simulink model "DiffDrive_Sim"  (R2022b)
settings: Solver=FixedStepAuto  StartTime=0.0  StopTime=120  FixedStep=Ts  RelTol=1e-3
values from neighbouring files (symbols this model uses):
  encoder_cpr = 12    [load_model.m]
  max_turning_radius = 100    [load_model.m]
  motor_FF_factor = 1.0    (= 1)    [load_model.m]
  motor_gear = 1/75    (= 0.0133333333333)    [load_model.m]
  motor_tf = load('..\data\platform\TF_motor.mat').TF_MOT    [load_model.m]
  motor_Ts = 50e-3    (= 0.05)    [load_model.m]
  motor_vcc = 5.93    [load_model.m]
  motor_vel_max = 47.5    [load_model.m]
  PID_mot_vel_coeff = get_PID_coeff(PID_mot_vel, motor_Ts)    [load_model.m]
  Ts = 1e-3    (= 0.001)    [load_model.m]
  wheel_radius = 0.01625    [load_model.m]
  wheel_track = 0.125/2    (= 0.0625)    [load_model.m]
libraries: cstblocks x2
settings Model: Creator=alexr  LastModifiedBy=alexr

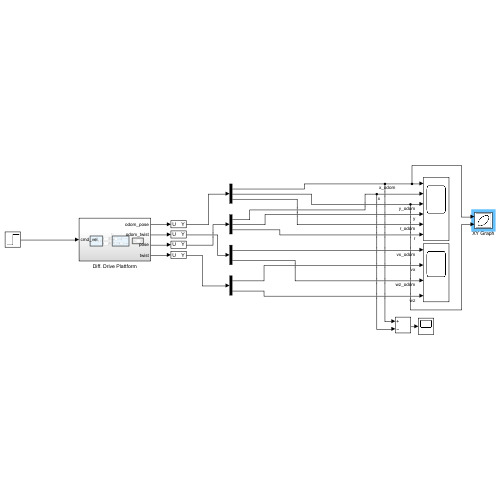
[thumbnail: Simulink's stored preview of the top-level diagram]
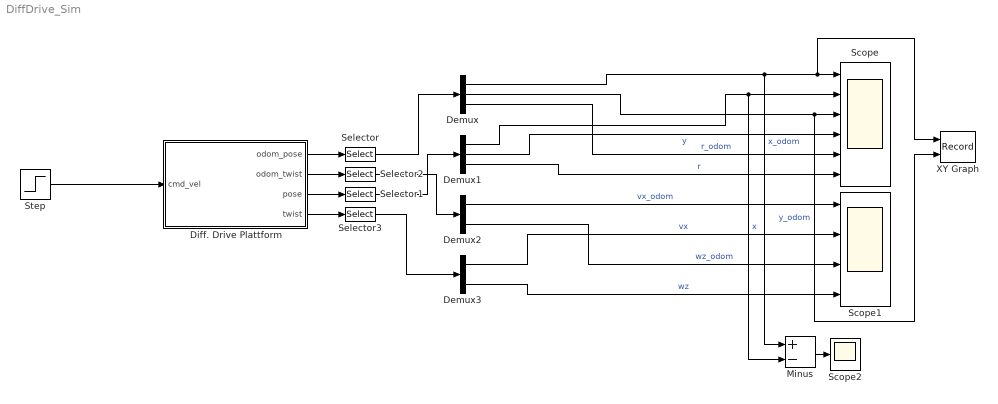
== system DiffDrive_Sim ==
  Demux : Demux  Outputs=3
  Demux1 : Demux  Outputs=3
  Demux2 : Demux  Outputs=2
  Demux3 : Demux  Outputs=2
  Diff. Drive Plattform : Subsystem
  Minus : Sum  Inputs=+-
  Scope : Scope  NumInputPorts=6
  Scope1 : Scope  NumInputPorts=4
  Scope2 : Scope
  Selector : Selector  InputPortWidth=6  IndexOptions=Index vector (dialog)  Indices=[1 2 6]  OutputSizes=1
  Selector1 : Selector  InputPortWidth=6  IndexOptions=Index vector (dialog)  Indices=[1 2 6]  OutputSizes=1
  Selector2 : Selector  InputPortWidth=6  IndexOptions=Index vector (dialog)  Indices=[1 6]  OutputSizes=1
  Selector3 : Selector  InputPortWidth=6  IndexOptions=Index vector (dialog)  Indices=[1 6]  OutputSizes=1
  Step : Step  After=[.1 0 0 0 0 .5]'  SampleTime=0
  XY Graph : Record  FileSettingsInternal="{\"entries\":[{\"content\":{\"excelSettings\":{\"content\":{},\"type\":\"Streamout.ExcelSettings\"}},\"type\":\"Streamout.FileSettingStorage\",\"uuid\":\"8a958047-305f-4305-a06c-71493970eef4\"}],\"packageUris\":[\"http://schema.mathworks.com/mf0/streamout_blocks/R2020a\"],\"version\":\"1.0\"}"  Layout=[1 1]  SignalsInternal="{\"entries\":[{\"content\":{\"signals\":[{\"content\":{\"blockPath\":[\"DiffDrive_Sim/XY Graph\"],\"channel\":[],\"dimensions\":[1,1],\"domain\":\"DiffDrive_Sim/XY Graph\",\"lineColor\":\"#a2142f\",\"plots\":[1],\"port\":1,\"sid\":[\"\"],\"signalID\":1115,\"signalName\":\"x_odom\"},\"type\":\"RecordBlkView.Signal\",\"uuid\":\"f2926a7d-a479-4f30-9233-b48412fcda20\"},{\"content\":{\"blockPath\":[\"DiffDrive_Sim/XY Graph\"],\"channel\":[],\"dimensions\":[1,1],\"domain\":\"DiffDrive_Sim/XY Graph\",\"lineColor\":\"#139fff\",\"plots\":[1],\"port\":2,\"sid\":[\"\"],\"signalID\":1119,\"signalName\":\"y_odom\"},\"type\":\"RecordBlkView.Signal\",\"uuid\":\"88293d54-0842-49fd-9493-97809c72c41e\"}]},\"type\":\"RecordBlkView.InputSignals\",\"uuid\":\"56c78d2d-7b90-4c9a-a923-81b59751f0cd\"}],\"packageUris\":[\"http://schema.mathworks.com/mf0/streamout_blocks/R2020a\"],\"version\":\"1.0\"}"  VisualizationBindings="{\"xyplotplugin\":{\"info\":[{\"series\":[{\"bindingParametersList\":[{\"parameter\":\"X-Axis\",\"signalID\":1115,\"signalName\":\"x_odom\"},{\"parameter\":\"Y-Axis\",\"signalID\":1119,\"signalName\":\"y_odom\"}],\"seriesID\":46262}],\"subplotID\":1}]}}"  CompatibilityTag=XY
  wires:
  Diff. Drive Plattform/1(odom_pose) -> Selector/1
  Diff. Drive Plattform/3(pose) -> Selector1/1
  Diff. Drive Plattform/2(odom_twist) -> Selector2/1
  Diff. Drive Plattform/4(twist) -> Selector3/1
  Selector/1 -> Demux/1
  Selector2/1 -> Demux2/1
  Selector1/1 -> Demux1/1
  Selector3/1 -> Demux3/1
  Demux/1 -> Minus/1, XY Graph/1, Scope/1  "x_odom"
  Demux1/1 -> Minus/2, Scope/2  "x"
  Demux/2 -> XY Graph/2, Scope/3  "y_odom"
  Demux1/2 -> Scope/4  "y"
  Demux/3 -> Scope/5  "r_odom"
  Demux1/3 -> Scope/6  "r"
  Demux2/1 -> Scope1/1  "vx_odom"
  Demux3/1 -> Scope1/2  "vx"
  Demux2/2 -> Scope1/3  "wz_odom"
  Demux3/2 -> Scope1/4  "wz"
  Step/1 -> Diff. Drive Plattform/1(cmd_vel)
  Minus/1 -> Scope2/1

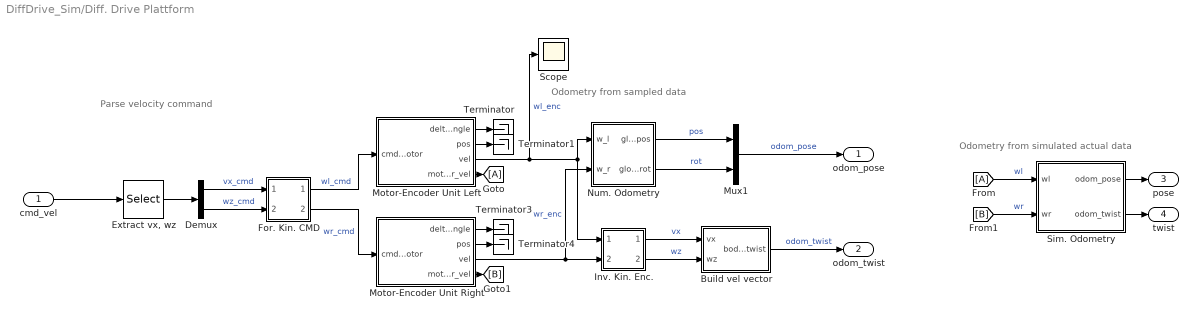
== system DiffDrive_Sim/Diff. Drive Plattform ==
  note: Odometry from simulated actual data
  note: Parse velocity command
  note: Odometry from sampled data
  cmd_vel : Inport
  Build vel vector : Subsystem
  Demux : Demux  Outputs=2
  "Extract vx, wz" : Selector  InputPortWidth=6  IndexOptions=Index vector (dialog)  Indices=[1 6]  OutputSizes=1
  For. Kin. CMD : Subsystem  mask{par_wheel_track=wheel_track, par_wheel_radius=wheel_radius}
      mask prompts: par_wheel_track "Wheel track"; par_wheel_radius "Wheel radius"
      mask DialogControl DescGroupVar Prompt: Forward Kinematics of a Differential Drive Robot
      mask DialogControl DescTextVar Prompt: Transforms body data to wheels
  From : From
  Goto : Goto
  Inv. Kin. Enc. : Subsystem  mask{par_wheel_track=wheel_track, par_wheel_radius=wheel_radius}
      mask prompts: par_wheel_track "Wheel track"; par_wheel_radius "Wheel radius"
      mask DialogControl DescGroupVar Prompt: Inverse Kinematics of a Differential Drive Robot
      mask DialogControl DescTextVar Prompt: Transforms wheel data to body data.
  Motor-Encoder Unit Left : Subsystem
  Motor-Encoder Unit Right : Subsystem
  Mux1 : Mux  Inputs=2
  Num. Odometry : Subsystem  mask{par_wheel_track=wheel_track, par_wheel_radius=wheel_radius, par_max_turning_radius=max_turning_radius, par_Ts=motor_Ts, par_fast=on}
      mask prompts: par_wheel_track "Wheel track"; par_wheel_radius "Wheel radius"; par_max_turning_radius "Maximum turning radius"; par_Ts "Sample time"; par_fast "Use approximation for position updates."
      mask DialogControl DescGroupVar Prompt: Odometry computation of a Differential Drive Robot
      mask DialogControl DescTextVar Prompt: Calculates the global position and orientation from encoder data.
      mask DialogControl par_max_turning_radius Tooltip: Used for exact computation only
      mask DialogControl par_fast Tooltip: Faster, but less accurate.
  Scope : Scope
  Sim. Odometry : Subsystem
  Terminator{,1,3..4} (4 alike) : Terminator
  odom_pose : Outport
  odom_twist : Outport  Port=2
  pose : Outport  Port=3
  twist : Outport  Port=4
  wires:
  Build vel vector/1(body_twist) -> odom_twist/1  "odom_twist"
  From/1 -> Sim. Odometry/1(wl)  "wl"
  Mux1/1 -> odom_pose/1  "odom_pose"
  Sim. Odometry/2(odom_twist) -> twist/1
  Motor-Encoder Unit Right/4(motor_vel) -> [B]
  Motor-Encoder Unit Left/4(motor_vel) -> Goto/1
  [B] -> Sim. Odometry/2(wr)  "wr"
  Num. Odometry/2(glob_rot) -> Mux1/2  "rot"
  Inv. Kin. Enc./2(w_z) -> Build vel vector/2(wz)  "wz"
  Motor-Encoder Unit Right/1(delta_angle) -> Terminator3/1
  Motor-Encoder Unit Left/1(delta_angle) -> Terminator/1
  "Extract vx, wz"/1 -> Demux/1
  Motor-Encoder Unit Left/2(pos) -> Terminator1/1
  For. Kin. CMD/2(w_r) -> Motor-Encoder Unit Right/1(cmd_vel_motor)  "wr_cmd"
  Demux/1 -> For. Kin. CMD/1(v_x)  "vx_cmd"
  cmd_vel/1 -> "Extract vx, wz"/1
  Demux/2 -> For. Kin. CMD/2(w_z)  "wz_cmd"
  Sim. Odometry/1(odom_pose) -> pose/1
  For. Kin. CMD/1(w_l) -> Motor-Encoder Unit Left/1(cmd_vel_motor)  "wl_cmd"
  Motor-Encoder Unit Left/3(vel) -> Scope/1, Inv. Kin. Enc./1(w_l), Num. Odometry/1(w_l)  "wl_enc"
  Motor-Encoder Unit Right/3(vel) -> Num. Odometry/2(w_r), Inv. Kin. Enc./2(w_r)  "wr_enc"
  Motor-Encoder Unit Right/2(pos) -> Terminator4/1
  Num. Odometry/1(glob_pos) -> Mux1/1  "pos"
  Inv. Kin. Enc./1(v_x) -> Build vel vector/1(vx)  "vx"

== system DiffDrive_Sim/Diff. Drive Plattform/Build vel vector ==
  vx : Inport
  wz : Inport  Port=2
  Demux1 : Demux
  Mux : Mux  Inputs=6
  Zeros : Constant  Value=[0,0,0,0]
  body_twist : Outport
  wires:
  Demux1/1 -> Mux/2  "vy"
  Zeros/1 -> Demux1/1
  wz/1 -> Mux/6
  Demux1/4 -> Mux/5  "wy"
  Demux1/2 -> Mux/3  "vz"
  Demux1/3 -> Mux/4  "wx"
  Mux/1 -> body_twist/1  "body_twist"
  vx/1 -> Mux/1

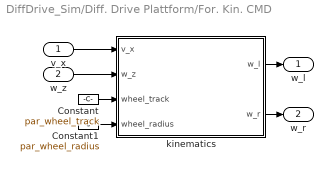
== system DiffDrive_Sim/Diff. Drive Plattform/For. Kin. CMD ==
  v_x : Inport
  w_z : Inport  Port=2
  Constant : Constant  Value=par_wheel_track
  Constant1 : Constant  Value=par_wheel_radius
  "kinematics " : MATLAB Function  TreatAsAtomicUnit=on
  w_l : Outport
  w_r : Outport  Port=2
  wires:
  w_z/1 -> "kinematics "/2(w_z)
  "kinematics "/1(w_l) -> w_l/1
  "kinematics "/2(w_r) -> w_r/1
  v_x/1 -> "kinematics "/1(v_x)
  Constant1/1 -> "kinematics "/4(wheel_radius)
  Constant/1 -> "kinematics "/3(wheel_track)

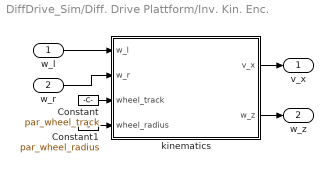
== system DiffDrive_Sim/Diff. Drive Plattform/Inv. Kin. Enc. ==
  w_l : Inport
  w_r : Inport  Port=2
  Constant : Constant  Value=par_wheel_track
  Constant1 : Constant  Value=par_wheel_radius
  kinematics : MATLAB Function  TreatAsAtomicUnit=on
  v_x : Outport
  w_z : Outport  Port=2
  wires:
  Constant/1 -> kinematics/3(wheel_track)
  w_r/1 -> kinematics/2(w_r)
  Constant1/1 -> kinematics/4(wheel_radius)
  kinematics/2(w_z) -> w_z/1
  kinematics/1(v_x) -> v_x/1
  w_l/1 -> kinematics/1(w_l)

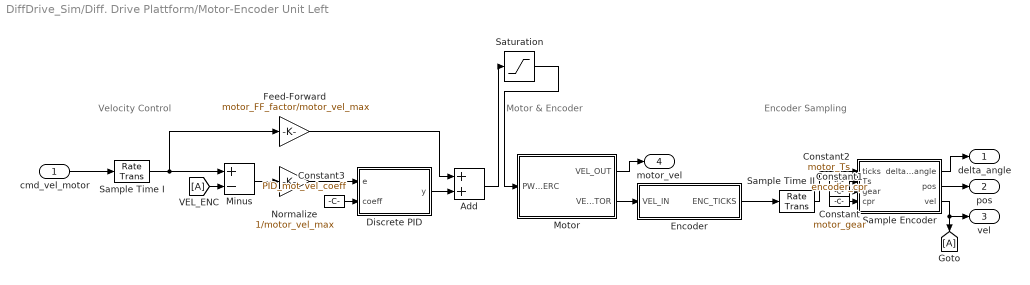
== system DiffDrive_Sim/Diff. Drive Plattform/Motor-Encoder Unit Left ==
  note: Encoder Sampling
  note: Motor & Encoder
  note: Velocity Control
  cmd_vel_motor : Inport
  Add : Sum
  Constant : Constant  Value=motor_gear
  Constant1 : Constant  Value=encoder_cpr
  Constant2 : Constant  Value=motor_Ts
  Constant3 : Constant  Value=PID_mot_vel_coeff
  Discrete PID : MATLAB Function  TreatAsAtomicUnit=on
  Encoder : Subsystem  mask{par_cpr=encoder_cpr, par_noise_on=on, par_ampl=.5, par_mean=0, par_var=1, par_seed=0}
      mask prompts: par_cpr "CPR"; par_noise_on "Enable"; par_ampl "Amplitude"; par_mean "Mean"; par_var "Variance"; par_seed "Seed"
      mask DialogControl DescGroupVar Prompt: Simple Hall Encoder
      mask DialogControl DescTextVar Prompt: A model of a simple hall encoder quantizing the revolutions the input.
      mask DialogControl Container2 Prompt: Quantization noise
      mask DialogControl Control2 Prompt: Adds gaussean noise to the encoder data.
  Feed-Forward : Gain  Gain=motor_FF_factor/motor_vel_max
  Goto : Goto
  Minus : Sum  Inputs=+-
  Motor : Subsystem  mask{par_tf=motor_tf, par_vcc=motor_vcc, par_gear=motor_gear}
      mask prompts: par_tf "Transfer function"; par_vcc "Supply voltage"; par_gear "Gear ratio"
      mask DialogControl DescGroupVar Prompt: Simple geared DC Motor
      mask DialogControl DescTextVar Prompt: A simple DC motor model based only on the transfer function and the supply voltage of the motor.
  Normalize : Gain  Gain=1/motor_vel_max
  Sample Encoder : MATLAB Function  TreatAsAtomicUnit=on
  Sample Time I : RateTransition  OutPortSampleTime=motor_Ts
  Sample Time II : RateTransition  OutPortSampleTime=motor_Ts
  Saturation : Saturate  UpperLimit=1  LowerLimit=-1
  VEL_ENC : From
  delta_angle : Outport
  pos : Outport  Port=2
  vel : Outport  Port=3
  motor_vel : Outport  Port=4
  wires:
  Add/1 -> Saturation/1
  Normalize/1 -> Discrete PID/1(e)
  Sample Time II/1 -> Sample Encoder/1(ticks)
  Minus/1 -> Normalize/1
  Constant/1 -> Sample Encoder/3(gear)
  Sample Time I/1 -> Feed-Forward/1, Minus/1
  Discrete PID/1(y) -> Add/2
  Constant3/1 -> Discrete PID/2(coeff)
  Constant2/1 -> Sample Encoder/2(Ts)
  Motor/2(VEL_MOTOR) -> Encoder/1(VEL_IN)
  Constant1/1 -> Sample Encoder/4(cpr)
  Encoder/1(ENC_TICKS) -> Sample Time II/1
  Sample Encoder/1(delta_angle) -> delta_angle/1
  Feed-Forward/1 -> Add/1
  VEL_ENC/1 -> Minus/2
  Sample Encoder/3(vel) -> Goto/1, vel/1
  Sample Encoder/2(pos) -> pos/1
  Motor/1(VEL_OUT) -> motor_vel/1
  cmd_vel_motor/1 -> Sample Time I/1
  Saturation/1 -> Motor/1(PWM_PERC)

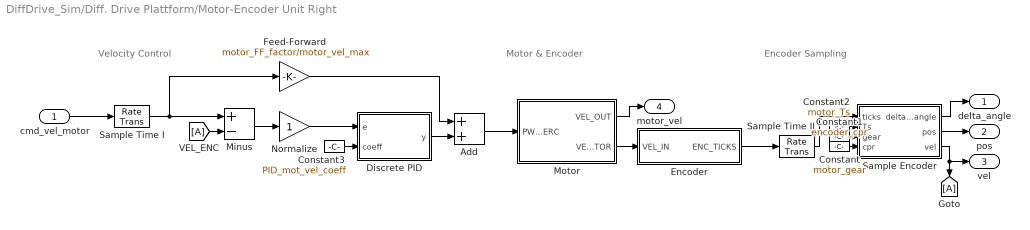
== system DiffDrive_Sim/Diff. Drive Plattform/Motor-Encoder Unit Right ==
  note: Encoder Sampling
  note: Motor & Encoder
  note: Velocity Control
  cmd_vel_motor : Inport
  Add : Sum
  Constant : Constant  Value=motor_gear
  Constant1 : Constant  Value=encoder_cpr
  Constant2 : Constant  Value=motor_Ts
  Constant3 : Constant  Value=PID_mot_vel_coeff
  Discrete PID : MATLAB Function  TreatAsAtomicUnit=on
  Encoder : Subsystem  mask{par_cpr=encoder_cpr, par_noise_on=on, par_ampl=1, par_mean=0, par_var=.5, par_seed=0}
      mask prompts: par_cpr "CPR"; par_noise_on "Enable"; par_ampl "Amplitude"; par_mean "Mean"; par_var "Variance"; par_seed "Seed"
      mask DialogControl DescGroupVar Prompt: Simple Hall Encoder
      mask DialogControl DescTextVar Prompt: A model of a simple hall encoder quantizing the revolutions the input.
      mask DialogControl Container2 Prompt: Quantization noise
      mask DialogControl Control2 Prompt: Adds gaussean noise to the encoder data.
  Feed-Forward : Gain  Gain=motor_FF_factor/motor_vel_max
  Goto : Goto
  Minus : Sum  Inputs=+-
  Motor : Subsystem  mask{par_tf=motor_tf, par_vcc=motor_vcc, par_gear=motor_gear}
      mask prompts: par_tf "Transfer function"; par_vcc "Supply voltage"; par_gear "Gear ratio"
      mask DialogControl DescGroupVar Prompt: Simple geared DC Motor
      mask DialogControl DescTextVar Prompt: A simple DC motor model based only on the transfer function and the supply voltage of the motor.
  Normalize : Gain
  Sample Encoder : MATLAB Function  TreatAsAtomicUnit=on
  Sample Time I : RateTransition  OutPortSampleTime=motor_Ts
  Sample Time II : RateTransition  OutPortSampleTime=motor_Ts
  VEL_ENC : From
  delta_angle : Outport
  pos : Outport  Port=2
  vel : Outport  Port=3
  motor_vel : Outport  Port=4
  wires:
  Add/1 -> Motor/1(PWM_PERC)
  Normalize/1 -> Discrete PID/1(e)
  Sample Time II/1 -> Sample Encoder/1(ticks)
  Minus/1 -> Normalize/1
  Constant/1 -> Sample Encoder/3(gear)
  Sample Time I/1 -> Feed-Forward/1, Minus/1
  Discrete PID/1(y) -> Add/2
  Constant3/1 -> Discrete PID/2(coeff)
  Constant2/1 -> Sample Encoder/2(Ts)
  Motor/2(VEL_MOTOR) -> Encoder/1(VEL_IN)
  Constant1/1 -> Sample Encoder/4(cpr)
  Encoder/1(ENC_TICKS) -> Sample Time II/1
  Sample Encoder/1(delta_angle) -> delta_angle/1
  Feed-Forward/1 -> Add/1
  VEL_ENC/1 -> Minus/2
  Sample Encoder/3(vel) -> Goto/1, vel/1
  Sample Encoder/2(pos) -> pos/1
  Motor/1(VEL_OUT) -> motor_vel/1
  cmd_vel_motor/1 -> Sample Time I/1

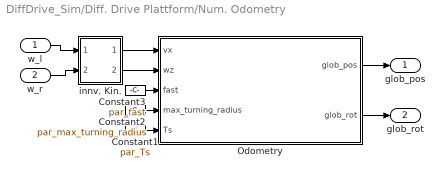
== system DiffDrive_Sim/Diff. Drive Plattform/Num. Odometry ==
  w_l : Inport
  w_r : Inport  Port=2
  Constant1 : Constant  Value=par_Ts
  Constant2 : Constant  Value=par_max_turning_radius
  Constant3 : Constant  Value=par_fast
  Odometry : MATLAB Function  TreatAsAtomicUnit=on
  innv. Kin. : Subsystem  mask{par_wheel_track=par_wheel_track, par_wheel_radius=par_wheel_radius}
      mask prompts: par_wheel_track "Wheel track"; par_wheel_radius "Wheel radius"
      mask DialogControl DescGroupVar Prompt: Inverse Kinematics of a Differential Drive Robot
      mask DialogControl DescTextVar Prompt: Transforms wheel data to body data.
  glob_pos : Outport
  glob_rot : Outport  Port=2
  wires:
  Constant2/1 -> Odometry/4(max_turning_radius)
  Odometry/1(glob_pos) -> glob_pos/1
  Odometry/2(glob_rot) -> glob_rot/1
  Constant3/1 -> Odometry/3(fast)
  w_l/1 -> innv. Kin./1(w_l)
  w_r/1 -> innv. Kin./2(w_r)
  innv. Kin./1(v_x) -> Odometry/1(vx)
  innv. Kin./2(w_z) -> Odometry/2(wz)
  Constant1/1 -> Odometry/5(Ts)

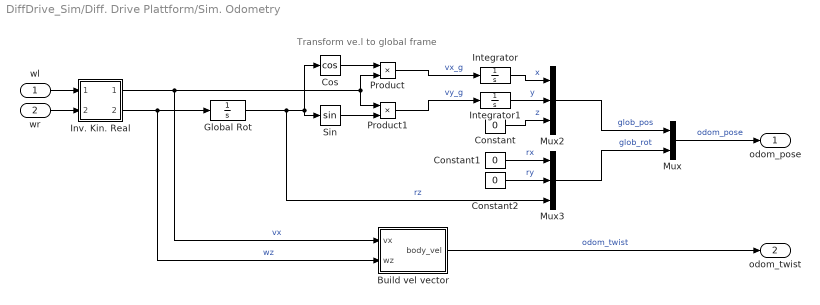
== system DiffDrive_Sim/Diff. Drive Plattform/Sim. Odometry ==
  note: Transform ve.l to global frame
  wl : Inport
  wr : Inport  Port=2
  Build vel vector : Subsystem
  Constant : Constant  Value=0
  Constant1 : Constant  Value=0
  Constant2 : Constant  Value=0
  Cos : Trigonometry  Operator=cos
  Global Rot : Integrator
  Integrator : Integrator
  Integrator1 : Integrator
  Inv. Kin. Real : Subsystem  mask{par_wheel_track=wheel_track, par_wheel_radius=wheel_radius}
      mask prompts: par_wheel_track "Wheel track"; par_wheel_radius "Wheel radius"
      mask DialogControl DescGroupVar Prompt: Inverse Kinematics of a Differential Drive Robot
      mask DialogControl DescTextVar Prompt: Transforms wheel data to body data.
  Mux : Mux  Inputs=2
  Mux2 : Mux  Inputs=3
  Mux3 : Mux  Inputs=3
  Product : Product
  Product1 : Product
  Sin : Trigonometry
  odom_pose : Outport
  odom_twist : Outport  Port=2
  wires:
  Integrator1/1 -> Mux2/2  "y"
  Product/1 -> Integrator/1  "vx_g"
  Constant/1 -> Mux2/3  "z"
  Constant1/1 -> Mux3/1  "rx"
  Inv. Kin. Real/1(v_x) -> Build vel vector/1(vx), Product/2, Product1/1  "vx"
  Global Rot/1 -> Mux3/3, Cos/1, Sin/1  "rz"
  Integrator/1 -> Mux2/1  "x"
  Cos/1 -> Product/1
  Inv. Kin. Real/2(w_z) -> Build vel vector/2(wz), Global Rot/1  "wz"
  Product1/1 -> Integrator1/1  "vy_g"
  Sin/1 -> Product1/2
  Constant2/1 -> Mux3/2  "ry"
  wr/1 -> Inv. Kin. Real/2(w_r)
  wl/1 -> Inv. Kin. Real/1(w_l)
  Mux2/1 -> Mux/1  "glob_pos"
  Mux3/1 -> Mux/2  "glob_rot"
  Mux/1 -> odom_pose/1  "odom_pose"
  Build vel vector/1(body_vel) -> odom_twist/1  "odom_twist"

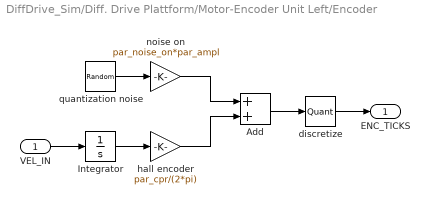
== system DiffDrive_Sim/Diff. Drive Plattform/Motor-Encoder Unit Left/Encoder ==
  VEL_IN : Inport
  Add : Sum
  Integrator : Integrator
  discretize : Quantizer  QuantizationInterval=1
  hall encoder : Gain  Gain=par_cpr/(2*pi)
  noise on : Gain  Gain=par_noise_on*par_ampl
  quantization noise : RandomNumber  Mean=par_mean  Variance=par_var  Seed=par_seed  SampleTime=Ts
  ENC_TICKS : Outport
  wires:
  VEL_IN/1 -> Integrator/1
  Integrator/1 -> hall encoder/1
  quantization noise/1 -> noise on/1
  Add/1 -> discretize/1
  hall encoder/1 -> Add/2
  discretize/1 -> ENC_TICKS/1
  noise on/1 -> Add/1

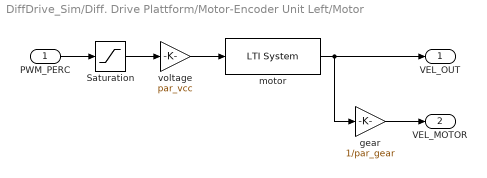
== system DiffDrive_Sim/Diff. Drive Plattform/Motor-Encoder Unit Left/Motor ==
  PWM_PERC : Inport
  Saturation : Saturate  UpperLimit=1  LowerLimit=-1
  gear : Gain  Gain=1/par_gear
  motor : cstblocks/LTI System  sys=par_tf  IC=[]
  voltage : Gain  Gain=par_vcc
  VEL_OUT : Outport
  VEL_MOTOR : Outport  Port=2
  wires:
  PWM_PERC/1 -> Saturation/1
  voltage/1 -> motor/1
  motor/1 -> gear/1, VEL_OUT/1
  Saturation/1 -> voltage/1
  gear/1 -> VEL_MOTOR/1

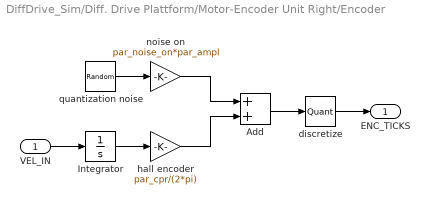
== system DiffDrive_Sim/Diff. Drive Plattform/Motor-Encoder Unit Right/Encoder ==
  VEL_IN : Inport
  Add : Sum
  Integrator : Integrator
  discretize : Quantizer  QuantizationInterval=1
  hall encoder : Gain  Gain=par_cpr/(2*pi)
  noise on : Gain  Gain=par_noise_on*par_ampl
  quantization noise : RandomNumber  Mean=par_mean  Variance=par_var  Seed=par_seed  SampleTime=Ts
  ENC_TICKS : Outport
  wires:
  VEL_IN/1 -> Integrator/1
  Integrator/1 -> hall encoder/1
  quantization noise/1 -> noise on/1
  Add/1 -> discretize/1
  hall encoder/1 -> Add/2
  discretize/1 -> ENC_TICKS/1
  noise on/1 -> Add/1

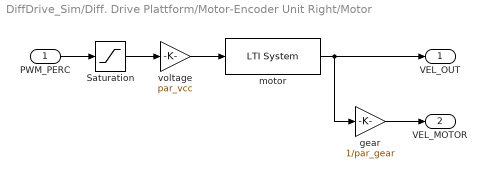
== system DiffDrive_Sim/Diff. Drive Plattform/Motor-Encoder Unit Right/Motor ==
  PWM_PERC : Inport
  Saturation : Saturate  UpperLimit=1  LowerLimit=-1
  gear : Gain  Gain=1/par_gear
  motor : cstblocks/LTI System  sys=par_tf  IC=[]
  voltage : Gain  Gain=par_vcc
  VEL_OUT : Outport
  VEL_MOTOR : Outport  Port=2
  wires:
  PWM_PERC/1 -> Saturation/1
  voltage/1 -> motor/1
  motor/1 -> gear/1, VEL_OUT/1
  Saturation/1 -> voltage/1
  gear/1 -> VEL_MOTOR/1

== system DiffDrive_Sim/Diff. Drive Plattform/Num. Odometry/innv. Kin. ==
  w_l : Inport
  w_r : Inport  Port=2
  Constant : Constant  Value=par_wheel_track
  Constant1 : Constant  Value=par_wheel_radius
  kinematics : MATLAB Function  TreatAsAtomicUnit=on
  v_x : Outport
  w_z : Outport  Port=2
  wires:
  Constant/1 -> kinematics/3(wheel_track)
  w_r/1 -> kinematics/2(w_r)
  Constant1/1 -> kinematics/4(wheel_radius)
  kinematics/2(w_z) -> w_z/1
  kinematics/1(v_x) -> v_x/1
  w_l/1 -> kinematics/1(w_l)

== system DiffDrive_Sim/Diff. Drive Plattform/Sim. Odometry/Build vel vector ==
  vx : Inport
  wz : Inport  Port=2
  Demux1 : Demux
  Mux : Mux  Inputs=6
  Zeros : Constant  Value=[0,0,0,0]
  body_vel : Outport
  wires:
  Demux1/1 -> Mux/2  "vy"
  Zeros/1 -> Demux1/1
  wz/1 -> Mux/6
  Demux1/4 -> Mux/5  "wy"
  Demux1/2 -> Mux/3  "vz"
  Demux1/3 -> Mux/4  "wx"
  Mux/1 -> body_vel/1  "body_vel"
  vx/1 -> Mux/1

== system DiffDrive_Sim/Diff. Drive Plattform/Sim. Odometry/Inv. Kin. Real ==
  w_l : Inport
  w_r : Inport  Port=2
  Constant : Constant  Value=par_wheel_track
  Constant1 : Constant  Value=par_wheel_radius
  kinematics : MATLAB Function  TreatAsAtomicUnit=on
  v_x : Outport
  w_z : Outport  Port=2
  wires:
  Constant/1 -> kinematics/3(wheel_track)
  w_r/1 -> kinematics/2(w_r)
  Constant1/1 -> kinematics/4(wheel_radius)
  kinematics/2(w_z) -> w_z/1
  kinematics/1(v_x) -> v_x/1
  w_l/1 -> kinematics/1(w_l)

== matlab function DiffDrive_Sim/Diff. Drive Plattform/Inv. Kin. Enc./kinematics ==
  data: w_l input; v_x output; w_r input; w_z output; wheel_track input; wheel_radius input
function [v_x, w_z] = inv_kin(w_l, w_r, wheel_track, wheel_radius)
    v_x = (w_l + w_r) * wheel_radius / 2;
    w_z = (w_r - w_l) * wheel_radius / (2 * wheel_track);

== matlab function DiffDrive_Sim/Diff. Drive Plattform/Motor-Encoder Unit Left/Discrete PID ==
  data: e input; y output; coeff input
function y = fcn(e, coeff)
    % Coefficients: k_y1, k_y2, k_e0, k_e1, k_e2
    % Buffer: y_{n-1}, y_{n-2}, e_{n-1}, e_{n-2}

    persistent buffer
    if isempty(buffer)
        buffer = [0, 0, 0, 0];
    end
    
    y = -coeff(1)*buffer(1) - coeff(2)*buffer(2) + coeff(3)*e + coeff(4)*buffer(3) + coeff(5)*buffer(4);

    buffer(2) = buffer(1);  % y_{n-1} -> y_{n-2}
    buffer(1) = y;          % y_{n} -> y_{n-1}
    buffer(4) = buffer(3);  % e_{n-1} -> e_{n-2}
    buffer(3) = e;          % e_{n} -> e_{n-1}

== matlab function DiffDrive_Sim/Diff. Drive Plattform/Motor-Encoder Unit Left/Sample Encoder ==
  data: delta_angle output; ticks input; pos output; vel output; Ts input; gear input; cpr input
function [delta_angle, pos, vel] = fcn(ticks, Ts, gear, cpr)
    persistent prev_ticks
    persistent angle
    if isempty(prev_ticks)
        prev_ticks = 0;
        angle = 0;
    end

    delta_angle = 2 * pi * (ticks - prev_ticks) * gear / cpr;
    prev_ticks = ticks;

    angle = angle + delta_angle;
    
    pos = angle;
    vel = delta_angle / Ts;

== matlab function DiffDrive_Sim/Diff. Drive Plattform/For. Kin. CMD/kinematics  ==
  data: v_x input; w_l output; w_z input; w_r output; wheel_track input; wheel_radius input
function [w_l, w_r]  = for_kin(v_x, w_z, wheel_track, wheel_radius)
    w_l = (v_x - w_z * wheel_track) /wheel_radius;
    w_r = (v_x + w_z * wheel_track) /wheel_radius;

== matlab function DiffDrive_Sim/Diff. Drive Plattform/Sim. Odometry/Inv. Kin. Real/kinematics ==
  data: w_l input; v_x output; w_r input; w_z output; wheel_track input; wheel_radius input
function [v_x, w_z] = inv_kin(w_l, w_r, wheel_track, wheel_radius)
    v_x = (w_l + w_r) * wheel_radius / 2;
    w_z = (w_r - w_l) * wheel_radius / (2 * wheel_track);

== matlab function DiffDrive_Sim/Diff. Drive Plattform/Motor-Encoder Unit Right/Discrete PID ==
  data: e input; y output; coeff input
function y = fcn(e, coeff)
    % Coefficients: k_y1, k_y2, k_e0, k_e1, k_e2
    % Buffer: y_{n-1}, y_{n-2}, e_{n-1}, e_{n-2}

    persistent buffer
    if isempty(buffer)
        buffer = [0, 0, 0, 0];
    end
    
    y = -coeff(1)*buffer(1) - coeff(2)*buffer(2) + coeff(3)*e + coeff(4)*buffer(3) + coeff(5)*buffer(4);

    if(y > 1)
        y = 1;
    elseif(y < -1)
        y = -1;
    end

    buffer(2) = buffer(1);  % y_{n-1} -> y_{n-2}
    buffer(1) = y;          % y_{n} -> y_{n-1}
    buffer(4) = buffer(3);  % e_{n-1} -> e_{n-2}
    buffer(3) = e;          % e_{n} -> e_{n-1}

== matlab function DiffDrive_Sim/Diff. Drive Plattform/Motor-Encoder Unit Right/Sample Encoder ==
  data: delta_angle output; ticks input; pos output; vel output; Ts input; gear input; cpr input
function [delta_angle, pos, vel] = fcn(ticks, Ts, gear, cpr)
    persistent prev_ticks
    if isempty(prev_ticks)
        prev_ticks = 0;
    end

    persistent angle
    if isempty(angle)
        angle = 0;
    end

    if isempty(prev_ticks)
        prev_ticks = 0;
    end

    delta_angle = 2 * pi * (ticks - prev_ticks) * gear / cpr;
    prev_ticks = ticks;

    angle = angle + delta_angle;


    
    pos = angle;
    vel = delta_angle / Ts;

== matlab function DiffDrive_Sim/Diff. Drive Plattform/Num. Odometry/Odometry ==
  data: vx input; wz input; glob_pos output; fast input; glob_rot output; max_turning_radius input; Ts input
function [glob_pos, glob_rot] = fcn(vx, wz, fast, max_turning_radius, Ts)
    persistent pos
    persistent rot
    if isempty(pos)
        pos = [0;0;0];
        rot = [0;0;0];
    end
        
    ds = vx * Ts;
    drot = wz * Ts;

    if(fast)
        pos(1) = pos(1) + ds * cos(rot(3) + drot/2);
        pos(2) = pos(2) + ds * sin(rot(3) + drot/2);
        rot(3) = rot(3) + drot;  
    else

        if(drot == 0)
            r_irc = max_turning_radius;
        else
            r_irc = ds / drot;
        end

        x = 0;
        y = 0;

        if(r_irc >= max_turning_radius || r_irc <= -max_turning_radius)
            x = ds;
        elseif(abs(r_irc) > 1e-3)
            x = r_irc * sin(drot);
            y = r_irc * (1 - cos(drot));
        end

        pos(1) = pos(1) + x*cos(rot(3)) - y * sin(rot(3));
        pos(2) = pos(2) + x*sin(rot(3)) + y * cos(rot(3));
        rot(3) = rot(3) + drot;     
    end

    glob_pos = pos;
    glob_rot = rot;

== matlab function DiffDrive_Sim/Diff. Drive Plattform/Num. Odometry/innv. Kin./kinematics ==
  data: w_l input; v_x output; w_r input; w_z output; wheel_track input; wheel_radius input
function [v_x, w_z] = inv_kin(w_l, w_r, wheel_track, wheel_radius)
    v_x = (w_l + w_r) * wheel_radius / 2;
    w_z = (w_r - w_l) * wheel_radius / (2 * wheel_track);
